simulink model "HANcoder_E407_TTA_Controller_v3"  (R2018b)
settings: Solver=FixedStepDiscrete  StartTime=0.0  StopTime=1  FixedStep=0.01  RelTol=1e-3
PreLoadFcn:
  | librarySetup
  | eval([bdroot,'_startup']) %Calling [modelName]_startup.m
values from neighbouring files (symbols this model uses):
  basic_cycle_duration_bc0 = TM_Reset_Board   + COMP_duration    (= 212)    [HANcoder_E407_TTA_Controller_v3_startup.m]
  basic_cycle_duration_bc1 = TM_Reset_Var_bc1 + COMP_duration    (= 288)    [HANcoder_E407_TTA_Controller_v3_startup.m]
  comm_delay_estimation1 = round(comm_delay_measured1*hardware_granularity/frequency_IRQ)    [HANcoder_E407_TTA_Controller_v3_startup.m]
  comm_delay_estimation2 = round(comm_delay_measured2*hardware_granularity/frequency_IRQ)    [HANcoder_E407_TTA_Controller_v3_startup.m]
  COMM_Period = 40    [HANcoder_E407_TTA_Controller_v3_startup.m]
  COMM_Phase1 = 5    [HANcoder_E407_TTA_Controller_v3_startup.m]
  COMM_Phase2 = 8    [HANcoder_E407_TTA_Controller_v3_startup.m]
  COMP_duration = 4    [HANcoder_E407_TTA_Controller_v3_startup.m]
  Controller1_Board = 1    [HANcoder_E407_TTA_Controller_v3_startup.m]
  Controller2_Board = 2    [HANcoder_E407_TTA_Controller_v3_startup.m]
  Controller3_Board = 3    [HANcoder_E407_TTA_Controller_v3_startup.m]
  delta_a_set = Simulink.Parameter    [HANcoder_E407_TTA_Controller_v3_startup.m]
  delta_f_set = Simulink.Parameter    [HANcoder_E407_TTA_Controller_v3_startup.m]
  delta_max = 1    [HANcoder_E407_TTA_Controller_v3_startup.m]
  delta_min = -1    [HANcoder_E407_TTA_Controller_v3_startup.m]
  delta_precision = 6    [HANcoder_E407_TTA_Controller_v3_startup.m]
  e_width = 0.1    [HANcoder_E407_TTA_Controller_v3_startup.m]
  frequency_IRQ = 100    [HANcoder_E407_TTA_Controller_v3_startup.m]
  HANtuneOverride = Simulink.Parameter    [HANcoder_E407_TTA_Controller_v3_startup.m]
  hardware_granularity = 1000000    [HANcoder_E407_TTA_Controller_v3_startup.m]
  I_a = 2.25    [HANcoder_E407_TTA_Controller_v3_startup.m]
  I_f = 2.25    [HANcoder_E407_TTA_Controller_v3_startup.m]
  idle_time_init = basic_cycle_duration_bc0 + basic_cycle_duration_bc1    (= 500)    [HANcoder_E407_TTA_Controller_v3_startup.m]
  Input_Gen_Board = 4    [HANcoder_E407_TTA_Controller_v3_startup.m]
  LA_Clock_Gr = 1    [HANcoder_E407_TTA_Controller_v3_startup.m]
  LA_COMM_Err = 0    [HANcoder_E407_TTA_Controller_v3_startup.m]
  LA_MEX_Flag = 0    [HANcoder_E407_TTA_Controller_v3_startup.m]
  LA_Task_Act = 1    [HANcoder_E407_TTA_Controller_v3_startup.m]
  m_v = 100.0    (= 100)    [HANcoder_E407_TTA_Controller_v3_startup.m]
  Master_Role = 1    [HANcoder_E407_TTA_Controller_v3_startup.m]
  matrix_cycle_duration = basic_cycle_duration_bc0 + basic_cycle_duration_bc1    (= 500)    [HANcoder_E407_TTA_Controller_v3_startup.m]
  matrix_rows = 2    [HANcoder_E407_TTA_Controller_v3_startup.m]
  max_num_msgs_CAN1 = 2^Tx_bit_number-1    (= 7)    [HANcoder_E407_TTA_Controller_v3_startup.m]
  max_num_msgs_CAN2 = max_num_msgs_CAN1    (= 7)    [HANcoder_E407_TTA_Controller_v3_startup.m]
  OutControl1_ID = 23    [HANcoder_E407_TTA_Controller_v3_startup.m]
  OutControl2_ID = 24    [HANcoder_E407_TTA_Controller_v3_startup.m]
  OutEmulator_ID = 25    [HANcoder_E407_TTA_Controller_v3_startup.m]
  R_al = 0.10    (= 0.1)    [HANcoder_E407_TTA_Controller_v3_startup.m]
  R_ar = 0.10    (= 0.1)    [HANcoder_E407_TTA_Controller_v3_startup.m]
  R_fl = 0.10    (= 0.1)    [HANcoder_E407_TTA_Controller_v3_startup.m]
  R_fr = 0.10    (= 0.1)    [HANcoder_E407_TTA_Controller_v3_startup.m]
  SensorValues_ID = 22    [HANcoder_E407_TTA_Controller_v3_startup.m]
  SetValues_ID = 21    [HANcoder_E407_TTA_Controller_v3_startup.m]
  Slave_Role = 2    [HANcoder_E407_TTA_Controller_v3_startup.m]
  speed_k_d = Simulink.Parameter    [HANcoder_E407_TTA_Controller_v3_startup.m]
  speed_k_i = Simulink.Parameter    [HANcoder_E407_TTA_Controller_v3_startup.m]
  speed_k_p = Simulink.Parameter    [HANcoder_E407_TTA_Controller_v3_startup.m]
  speed_max = 10    [HANcoder_E407_TTA_Controller_v3_startup.m]
  speed_min = -10    [HANcoder_E407_TTA_Controller_v3_startup.m]
  speed_precision = 3    [HANcoder_E407_TTA_Controller_v3_startup.m]
  Sync_ID = 1    [HANcoder_E407_TTA_Controller_v3_startup.m]
  tau_max = 5    [HANcoder_E407_TTA_Controller_v3_startup.m]
  tau_min = -5    [HANcoder_E407_TTA_Controller_v3_startup.m]
  tau_range = abs(tau_max) + abs(tau_min)    [HANcoder_E407_TTA_Controller_v3_startup.m]
  theta_max = 2    [HANcoder_E407_TTA_Controller_v3_startup.m]
  theta_min = -2    [HANcoder_E407_TTA_Controller_v3_startup.m]
  theta_precision = 5    [HANcoder_E407_TTA_Controller_v3_startup.m]
  Tl_a = 0.6    [HANcoder_E407_TTA_Controller_v3_startup.m]
  Tl_f = 0.6    [HANcoder_E407_TTA_Controller_v3_startup.m]
  TM_Check_Output_Control1 = TM_COMM_Output_Control1 + COMM_duration    (= 188)    [HANcoder_E407_TTA_Controller_v3_startup.m]
  TM_Check_Output_Control2 = TM_COMM_Output_Control2 + COMM_duration    (= 232)    [HANcoder_E407_TTA_Controller_v3_startup.m]
  TM_Check_Output_Emulator = TM_COMM_Output_Emulator + COMM_duration    (= 280)    [HANcoder_E407_TTA_Controller_v3_startup.m]
  TM_Check_Sensor_Values = TM_COMM_Sensor_Values + COMM_duration    (= 132)    [HANcoder_E407_TTA_Controller_v3_startup.m]
  TM_Check_Set_Values = TM_COMM_Set_Values + COMM_duration    (= 88)    [HANcoder_E407_TTA_Controller_v3_startup.m]
  TM_Check_Sync = TM_COMM_Sync   + COMM_duration    (= 40)    [HANcoder_E407_TTA_Controller_v3_startup.m]
  TM_Check_TOuts = TM_Count_Vote3 + COMP_duration    (= 196)    [HANcoder_E407_TTA_Controller_v3_startup.m]
  TM_Check_Vote1 = TM_COMM_Vote1  + COMM_duration    (= 92)    [HANcoder_E407_TTA_Controller_v3_startup.m]
  TM_Check_Vote2 = TM_COMM_Vote2  + COMM_duration    (= 140)    [HANcoder_E407_TTA_Controller_v3_startup.m]
  TM_Check_Vote3 = TM_COMM_Vote3  + COMM_duration    (= 188)    [HANcoder_E407_TTA_Controller_v3_startup.m]
  TM_COMM_Output_Control1 = TM_Velocity + COMP_duration    (= 148)    [HANcoder_E407_TTA_Controller_v3_startup.m]
  TM_COMM_Output_Control2 = TM_Check_Output_Control1 + COMP_duration    (= 192)    [HANcoder_E407_TTA_Controller_v3_startup.m]
  TM_COMM_Output_Emulator = TM_TMR + COMP_duration    (= 240)    [HANcoder_E407_TTA_Controller_v3_startup.m]
  TM_COMM_Sensor_Values = TM_Check_Set_Values + COMP_duration    (= 92)    [HANcoder_E407_TTA_Controller_v3_startup.m]
  TM_COMM_Set_Values = TM_Update_LT + COMP_duration    (= 48)    [HANcoder_E407_TTA_Controller_v3_startup.m]
  TM_COMM_Sync = basic_cycle_start    (= 0)    [HANcoder_E407_TTA_Controller_v3_startup.m]
  TM_COMM_Vote1 = TM_Vote_Dec    + COMP_duration    (= 52)    [HANcoder_E407_TTA_Controller_v3_startup.m]
  TM_COMM_Vote2 = TM_Count_Vote1 + COMP_duration    (= 100)    [HANcoder_E407_TTA_Controller_v3_startup.m]
  TM_COMM_Vote3 = TM_Count_Vote2 + COMP_duration    (= 148)    [HANcoder_E407_TTA_Controller_v3_startup.m]
  TM_Count_Vote1 = TM_Check_Vote1 + COMP_duration    (= 96)    [HANcoder_E407_TTA_Controller_v3_startup.m]
  TM_Count_Vote2 = TM_Check_Vote2 + COMP_duration    (= 144)    [HANcoder_E407_TTA_Controller_v3_startup.m]
  TM_Count_Vote3 = TM_Check_Vote3 + COMP_duration    (= 192)    [HANcoder_E407_TTA_Controller_v3_startup.m]
  TM_Data_bc0 = TM_COMM_Sync    (= 0)    [HANcoder_E407_TTA_Controller_v3_startup.m]
  TM_Data_bc1 = TM_Data_bc0(1:3)    [HANcoder_E407_TTA_Controller_v3_startup.m]
  TM_New_Master = TM_Check_TOuts + COMP_duration    (= 200)    [HANcoder_E407_TTA_Controller_v3_startup.m]
  TM_Reset_Board = TM_Reset_Var   + COMP_duration    (= 208)    [HANcoder_E407_TTA_Controller_v3_startup.m]
  TM_Reset_Var = TM_New_Master  + COMP_duration    (= 204)    [HANcoder_E407_TTA_Controller_v3_startup.m]
  TM_Reset_Var_bc1 = TM_Check_Output_Emulator + COMP_duration    (= 284)    [HANcoder_E407_TTA_Controller_v3_startup.m]
  TM_Steer = TM_Check_Sensor_Values + COMP_duration    (= 136)    [HANcoder_E407_TTA_Controller_v3_startup.m]
  TM_TMR = TM_Check_Output_Control2 + COMP_duration    (= 236)    [HANcoder_E407_TTA_Controller_v3_startup.m]
  TM_Torque = TM_Steer + COMP_duration    (= 140)    [HANcoder_E407_TTA_Controller_v3_startup.m]
  TM_Type_bc0 = COMM    (= 0)    [HANcoder_E407_TTA_Controller_v3_startup.m]
  TM_Type_bc1 = TM_Type_bc0(1:3)    [HANcoder_E407_TTA_Controller_v3_startup.m]
  TM_Update_LT = TM_Check_Sync  + COMP_duration    (= 44)    [HANcoder_E407_TTA_Controller_v3_startup.m]
  TM_Velocity = TM_Torque + COMP_duration    (= 144)    [HANcoder_E407_TTA_Controller_v3_startup.m]
  TM_Vote_Dec = TM_Update_LT   + COMP_duration    (= 48)    [HANcoder_E407_TTA_Controller_v3_startup.m]
  torque_a_k_d = Simulink.Parameter    [HANcoder_E407_TTA_Controller_v3_startup.m]
  torque_a_k_i = Simulink.Parameter    [HANcoder_E407_TTA_Controller_v3_startup.m]
  torque_a_k_p = Simulink.Parameter    [HANcoder_E407_TTA_Controller_v3_startup.m]
  torque_f_k_d = Simulink.Parameter    [HANcoder_E407_TTA_Controller_v3_startup.m]
  torque_f_k_i = Simulink.Parameter    [HANcoder_E407_TTA_Controller_v3_startup.m]
  torque_f_k_p = Simulink.Parameter    [HANcoder_E407_TTA_Controller_v3_startup.m]
  torque_precision = 4    [HANcoder_E407_TTA_Controller_v3_startup.m]
  v_set = Simulink.Parameter    [HANcoder_E407_TTA_Controller_v3_startup.m]
  Vehicle_Em_Board = 5    [HANcoder_E407_TTA_Controller_v3_startup.m]
  Vote1_ID = 11    [HANcoder_E407_TTA_Controller_v3_startup.m]
  Vote2_ID = 12    [HANcoder_E407_TTA_Controller_v3_startup.m]
  Vote3_ID = 13    [HANcoder_E407_TTA_Controller_v3_startup.m]
undefined symbols (not defined in the file or in its folder): A0, A1, A2, A3, A4, CON2
libraries: hdlsllib x352, HANcoder_STM32_Target x25, simulink x3, simulink_extras x1
(part 6 of 32)

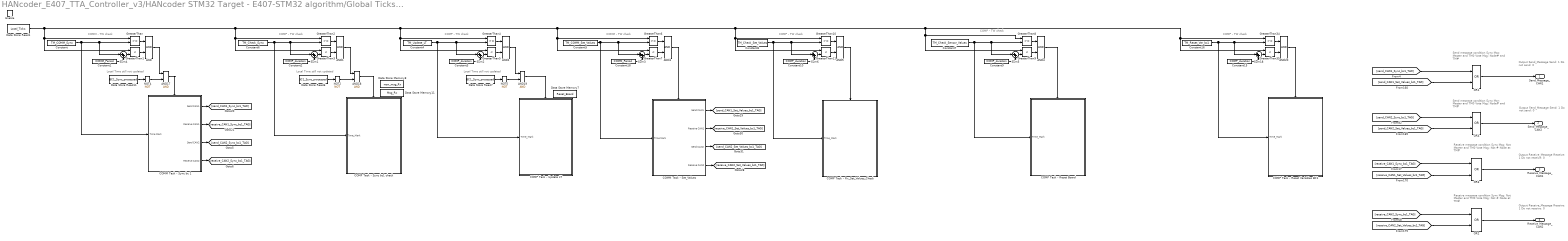
== system HANcoder_E407_TTA_Controller_v3/HANcoder STM32 Target - E407-STM32 algorithm/Global Ticks Increment/CAN Management/Matrix Cycle Manager/Input Generator Matrix Cycle/input generator basic cycle 1 ==
  note: COMP - TW check
  note: COMM - TW check
  note: Local Time still not updated
  note: Local Time still not updated
  note: COMP - TW check
  note: Local Time still not updated
  note: COMP - TW check
  note: COMP - TW check
  note: COMM - TW check
  note: Receive message condition
      | Sync Msg: Not Master and TM0
      | Vote Msg: Not # Node at TM#
  note: Send message condition
      | Sync Msg: Master and TM0
      | Vote Msg: Node# and TM#
  note: Output Send_Message
      | Send: 1
      | Do not send: 0
  note: Output Receive_Message
      | Receive: 1
      | Do not receive: 0
  note: Output Receive_Message
      | Receive: 1
      | Do not receive: 0
  note: Output Send_Message
      | Send: 1
      | Do not send: 0
  note: Send message condition
      | Sync Msg: Master and TM0
      | Vote Msg: Node# and TM#
  note: Receive message condition
      | Sync Msg: Not Master and TM0
      | Vote Msg: Not # Node at TM#
  note: COMP - TW check
  Enable : EnablePort
  AND{,1..5,17..20} (10 alike) : Logic  IconShape=distinctive  AllPortsSameDT=off  OutDataTypeStr=boolean
  COMM Task - Set_Values : Subsystem
  COMM Task - Sync bc 1 : Subsystem
  COMP Task - Reset Board : Subsystem
  COMP Task - Reset Variables BC1 : Subsystem
  COMP Task - Rx_Set_Values_Check : Subsystem
  COMP Task - Sync bc1 check : Subsystem
  COMP Task - Update LT : Subsystem
  Constant : Constant  Value=TM_COMM_Sync
  Constant1 : Constant  Value=COMM_Period
  Constant{2..3,9..10,15} (5 alike) : Constant  Value=COMP_duration
  Constant16 : Constant  Value=TM_Reset_Var_bc1
  Constant18 : Constant  Value=COMM_Period
  Constant4 : Constant  Value=TM_Update_LT
  Constant5 : Constant  Value=TM_COMM_Set_Values
  Constant6 : Constant  Value=TM_Check_Sync
  Constant7 : Constant  Value=TM_Check_Sensor_Values
  Constant8 : Constant  Value=TM_Check_Set_Values
  Data Store Memory11 : DataStoreMemory  DataStoreName=Msg_Rx  ReadBeforeWriteMsg=warning  WriteAfterWriteMsg=warning  WriteAfterReadMsg=warning  ShowAdditionalParam=off  OutDataTypeStr=Bus: msg_buffer_type
  Data Store Memory7 : DataStoreMemory  DataStoreName=Reset_Board  ReadBeforeWriteMsg=warning  WriteAfterWriteMsg=warning  WriteAfterReadMsg=warning  ShowAdditionalParam=off  OutDataTypeStr=boolean
  Data Store Memory8 : DataStoreMemory  DataStoreName=new_msg_Rx  ReadBeforeWriteMsg=warning  WriteAfterWriteMsg=warning  WriteAfterReadMsg=warning  ShowAdditionalParam=off
  Data Store Read1 : DataStoreRead  DataStoreName=Local_Ticks
  Data Store Read11 : DataStoreRead  DataStoreName=BC1_Sync_processed
  Data Store Read6 : DataStoreRead  DataStoreName=BC1_Sync_processed
  Data Store Read7 : DataStoreRead  DataStoreName=BC1_Sync_processed
  GreaterThan{,2,4,6,8,10,34} (7 alike) : RelationalOperator  OutDataTypeStr=boolean  RndMeth=Simplest
  GreaterThan{1,3,5,7,9,11,35} (7 alike) : RelationalOperator  Operator=<  OutDataTypeStr=boolean  RndMeth=Simplest
  NOT2 : Logic  Operator=NOT  IconShape=distinctive  AllPortsSameDT=off  OutDataTypeStr=boolean
  NOT4 : Logic  Operator=NOT  IconShape=distinctive  AllPortsSameDT=off  OutDataTypeStr=boolean
  NOT5 : Logic  Operator=NOT  IconShape=distinctive  AllPortsSameDT=off  OutDataTypeStr=boolean
  OR{1..4} (4 alike) : Logic  Operator=OR  IconShape=distinctive  AllPortsSameDT=off  OutDataTypeStr=boolean
  Sum{1..6,18} (7 alike) : Sum  Inputs=|++
  Send_Message_CAN1 : Outport  OutputWhenDisabled=reset  InitialOutput=0
  Send_Message_CAN2 : Outport  Port=2  OutputWhenDisabled=reset  InitialOutput=0
  Receive_Message_CAN1 : Outport  Port=3  OutputWhenDisabled=reset  InitialOutput=0
  Receive_Message_CAN2 : Outport  Port=4  OutputWhenDisabled=reset  InitialOutput=0
  wires:
  AND20/1 -> COMP Task - Reset Variables BC1/Enable
  GreaterThan34/1 -> AND20/1
  Sum18/1 -> GreaterThan35/2
  Constant15/1 -> Sum18/2
  Constant16/1 -> COMP Task - Reset Variables BC1/1(Time_Mark), GreaterThan34/2, Sum18/1
  GreaterThan35/1 -> AND20/2
  COMM Task - Set_Values/4(Receive CAN2) -> [receive_CAN2_Set_Values_bc1_TAG]
  COMM Task - Set_Values/3(Send CAN2) -> [send_CAN2_Set_Values_bc1_TAG]
  COMM Task - Set_Values/2(Receive CAN1) -> [receive_CAN1_Set_Values_bc1_TAG]
  COMM Task - Set_Values/1(Send CAN1) -> [send_CAN1_Set_Values_bc1_TAG]
  GreaterThan5/1 -> AND2/2
  Sum2/1 -> GreaterThan5/2
  NOT5/1 -> AND19/2
  COMM Task - Sync bc 1/3(Send CAN2) -> [send_CAN2_Sync_bc1_TAG]
  Sum1/1 -> GreaterThan3/2
  Constant6/1 -> Sum1/1, GreaterThan2/2, COMP Task - Sync bc1 check/1(Time_Mark)
  GreaterThan7/1 -> AND3/2
  Constant2/1 -> Sum1/2
  GreaterThan3/1 -> AND1/2
  GreaterThan2/1 -> AND1/1
  GreaterThan9/1 -> AND4/2
  GreaterThan8/1 -> AND4/1
  GreaterThan6/1 -> AND3/1
  Sum4/1 -> GreaterThan1/2
  Sum5/1 -> GreaterThan9/2
  Constant4/1 -> COMP Task - Update LT/1(Time_Mark), GreaterThan4/2, Sum2/1
  Sum3/1 -> GreaterThan7/2
  Constant7/1 -> COMP Task - Reset Board/1(Time_Mark), GreaterThan8/2, Sum5/1
  Constant3/1 -> Sum2/2
  AND/1 -> AND17/1
  Constant18/1 -> Sum3/2
  Constant5/1 -> Sum3/1, GreaterThan6/2, COMM Task - Set_Values/1(Time Mark)
  Constant/1 -> GreaterThan/2, Sum4/1, COMM Task - Sync bc 1/1(Time Mark)
  GreaterThan/1 -> AND/1
  GreaterThan1/1 -> AND/2
  NOT4/1 -> AND17/2
  Data Store Read6/1 -> NOT2/1
  AND2/1 -> AND19/1
  AND17/1 -> COMM Task - Sync bc 1/Enable
  Data Store Read11/1 -> NOT4/1
  AND1/1 -> AND18/1
  AND18/1 -> COMP Task - Sync bc1 check/Enable
  AND3/1 -> COMM Task - Set_Values/Enable
  GreaterThan4/1 -> AND2/1
  Data Store Read7/1 -> NOT5/1
  Constant9/1 -> Sum5/2
  NOT2/1 -> AND18/2
  AND4/1 -> COMP Task - Reset Board/Enable
  AND19/1 -> COMP Task - Update LT/Enable
  COMM Task - Sync bc 1/4(Receive CAN2) -> [receive_CAN2_Sync_bc1_TAG]
  COMM Task - Sync bc 1/2(Receive CAN1) -> [receive_CAN1_Sync_bc1_TAG]
  COMM Task - Sync bc 1/1(Send CAN1) -> [send_CAN1_Sync_bc1_TAG]
  Constant1/1 -> Sum4/2
  [receive_CAN2_Set_Values_bc1_TAG] -> OR2/2
  [receive_CAN2_Sync_bc1_TAG] -> OR2/1
  [receive_CAN1_Set_Values_bc1_TAG] -> OR3/2
  [receive_CAN1_Sync_bc1_TAG] -> OR3/1
  [send_CAN2_Set_Values_bc1_TAG] -> OR4/2
  [send_CAN2_Sync_bc1_TAG] -> OR4/1
  [send_CAN1_Set_Values_bc1_TAG] -> OR1/2
  [send_CAN1_Sync_bc1_TAG] -> OR1/1
  OR3/1 -> Receive_Message_CAN1/1
  OR4/1 -> Send_Message_CAN2/1
  OR2/1 -> Receive_Message_CAN2/1
  OR1/1 -> Send_Message_CAN1/1
  Constant8/1 -> COMP Task - Rx_Set_Values_Check/1(Time_Mark), Sum6/1, GreaterThan10/2
  GreaterThan10/1 -> AND5/1
  Data Store Read1/1 -> GreaterThan1/1, GreaterThan/1, GreaterThan3/1, GreaterThan2/1, GreaterThan5/1, GreaterThan4/1, GreaterThan7/1, GreaterThan6/1, GreaterThan35/1, GreaterThan34/1, GreaterThan9/1, GreaterThan8/1, GreaterThan11/1, GreaterThan10/1
  GreaterThan11/1 -> AND5/2
  Constant10/1 -> Sum6/2
  Sum6/1 -> GreaterThan11/2
  AND5/1 -> COMP Task - Rx_Set_Values_Check/Enable

== system HANcoder_E407_TTA_Controller_v3/HANcoder STM32 Target - E407-STM32 algorithm/Global Ticks Increment/CAN Management/Matrix Cycle Manager/Input Generator Matrix Cycle/msg_count_DEBUG observer ==
  Data Store Read24 : DataStoreRead  DataStoreName=msg_count_DEBUG
  Terminator : Terminator
  wires:
  Data Store Read24/1 -> Terminator/1  "msg_count_DEBUG_ing_s"

== system HANcoder_E407_TTA_Controller_v3/HANcoder STM32 Target - E407-STM32 algorithm/Global Ticks Increment/CAN Management/Matrix Cycle Manager/Vehicle Emulator Matrix Cycle/Matrix_Cycle_Observation_DEBUG ==
  Data Store Read : DataStoreRead  DataStoreName=Master_ID
  Data Store Read1 : DataStoreRead  DataStoreName=Role_ID
  Data Store Read10 : DataStoreRead  DataStoreName=BC1_Sync_processed
  Data Store Read2 : DataStoreRead  DataStoreName=BC0_Sync_processed
  Terminator{,1..2,12} (4 alike) : Terminator
  wires:
  Data Store Read1/1 -> Terminator/1  "Role_ID_vem_s"
  Data Store Read10/1 -> Terminator12/1  "BC1_sync_processed_vem__s"
  Data Store Read2/1 -> Terminator2/1  "BC0_sync_processed_vem__s"
  Data Store Read/1 -> Terminator1/1  "Master_ID_vem_s"

== system HANcoder_E407_TTA_Controller_v3/HANcoder STM32 Target - E407-STM32 algorithm/Global Ticks Increment/CAN Management/Matrix Cycle Manager/Vehicle Emulator Matrix Cycle/msg_count_DEBUG observer ==
  Data Store Read24 : DataStoreRead  DataStoreName=msg_count_DEBUG
  Terminator : Terminator
  wires:
  Data Store Read24/1 -> Terminator/1  "msg_count_DEBUG_vem_s"

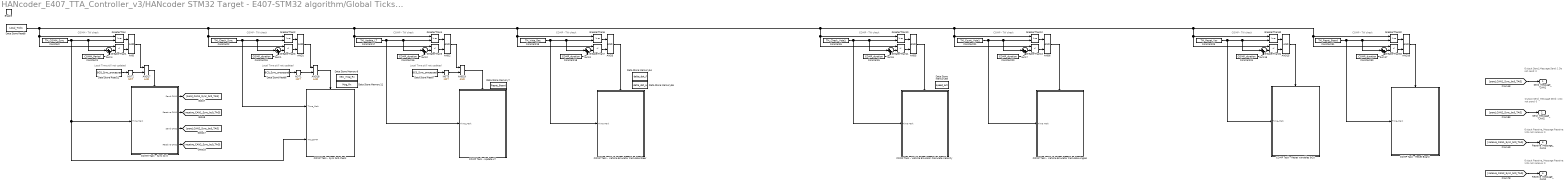
== system HANcoder_E407_TTA_Controller_v3/HANcoder STM32 Target - E407-STM32 algorithm/Global Ticks Increment/CAN Management/Matrix Cycle Manager/Vehicle Emulator Matrix Cycle/vehicle emulator basic cycle 0 ==
  note: Output Send_Message
      | Send: 1
      | Do not send: 0
  note: Output Receive_Message
      | Receive: 1
      | Do not receive: 0
  note: Output Send_Message
      | Send: 1
      | Do not send: 0
  note: Output Receive_Message
      | Receive: 1
      | Do not receive: 0
  note: COMM - TW check
  note: COMP - TW check
  note: COMP - TW check
  note: COMP - TW check
  note: COMP - TW check
  note: COMP - TW check
  note: COMP - TW check
  note: COMP - TW check
  note: Local Time still not updated
  note: Local Time still not updated
  note: Local Time still not updated
  Enable : EnablePort  PropagateVarSize=During execution
  AND{,1..3,5..6,15..19} (11 alike) : Logic  IconShape=distinctive  AllPortsSameDT=off  OutDataTypeStr=boolean
  COMM Task - Sync bc 0 : Subsystem
  COMP Task - Reset Board : Subsystem
  COMP Task - Reset Variables BC0 : Subsystem
  COMP Task - Sync bc0 check : Subsystem
  COMP Task - Update LT : Subsystem
  COMP Task - Vehicle Emulator Calculate Angles : Subsystem
  COMP Task - Vehicle Emulator Calculate Steer : Subsystem
  COMP Task - Vehicle Emulator Calculate Velocity : Subsystem
  Constant : Constant  Value=TM_COMM_Sync
  Constant1 : Constant  Value=COMM_Period
  Constant{5,15..16,18,20,24,30} (7 alike) : Constant  Value=COMP_duration
  Constant17 : Constant  Value=TM_Update_LT
  Constant19 : Constant  Value=TM_Vote_Dec
  Constant2 : Constant  Value=TM_Check_Sync
  Constant21 : Constant  Value=TM_Count_Vote1
  Constant25 : Constant  Value=TM_Reset_Var
  Constant31 : Constant  Value=TM_Reset_Board
  Constant6 : Constant  Value=TM_Check_Vote1
  Data Store Memory11 : DataStoreMemory  DataStoreName=Msg_Rx  ReadBeforeWriteMsg=warning  WriteAfterWriteMsg=warning  WriteAfterReadMsg=warning  ShowAdditionalParam=off  OutDataTypeStr=Bus: msg_buffer_type
  Data Store Memory54 : DataStoreMemory  DataStoreName=delta_dot_f  ReadBeforeWriteMsg=warning  WriteAfterWriteMsg=warning  WriteAfterReadMsg=warning  ShowAdditionalParam=off
  Data Store Memory56 : DataStoreMemory  DataStoreName=delta_dot_a  ReadBeforeWriteMsg=warning  WriteAfterWriteMsg=warning  WriteAfterReadMsg=warning  ShowAdditionalParam=off
  Data Store Memory59 : DataStoreMemory  DataStoreName=speed_act  ReadBeforeWriteMsg=warning  WriteAfterWriteMsg=warning  WriteAfterReadMsg=warning  ShowAdditionalParam=off
  Data Store Memory7 : DataStoreMemory  DataStoreName=Reset_Board  ReadBeforeWriteMsg=warning  WriteAfterWriteMsg=warning  WriteAfterReadMsg=warning  ShowAdditionalParam=off  OutDataTypeStr=boolean
  Data Store Memory8 : DataStoreMemory  DataStoreName=new_msg_Rx  ReadBeforeWriteMsg=warning  WriteAfterWriteMsg=warning  WriteAfterReadMsg=warning  ShowAdditionalParam=off
  Data Store Read11 : DataStoreRead  DataStoreName=BC0_Sync_processed
  Data Store Read6 : DataStoreRead  DataStoreName=BC0_Sync_processed
  Data Store Read7 : DataStoreRead  DataStoreName=BC0_Sync_processed
  Data Store Read8 : DataStoreRead  DataStoreName=Local_Ticks
  GreaterThan{,2,4,6,10,12,30,32} (8 alike) : RelationalOperator  OutDataTypeStr=boolean  RndMeth=Simplest
  GreaterThan{1,3,5,7,11,13,31,33} (8 alike) : RelationalOperator  Operator=<  OutDataTypeStr=boolean  RndMeth=Simplest
  NOT1 : Logic  Operator=NOT  IconShape=distinctive  AllPortsSameDT=off  OutDataTypeStr=boolean
  NOT2 : Logic  Operator=NOT  IconShape=distinctive  AllPortsSameDT=off  OutDataTypeStr=boolean
  NOT3 : Logic  Operator=NOT  IconShape=distinctive  AllPortsSameDT=off  OutDataTypeStr=boolean
  Sum{1..4,6..7,16..17} (8 alike) : Sum  Inputs=|++
  Send_Message_CAN1 : Outport  OutputWhenDisabled=reset  InitialOutput=0
  Send_Message_CAN2 : Outport  Port=2  OutputWhenDisabled=reset  InitialOutput=0
  Receive_Message_CAN1 : Outport  Port=3  OutputWhenDisabled=reset  InitialOutput=0
  Receive_Message_CAN2 : Outport  Port=4  OutputWhenDisabled=reset  InitialOutput=0
  wires:
  COMM Task - Sync bc 0/1(Send CAN1) -> [send_CAN1_Sync_bc0_TAG]
  COMM Task - Sync bc 0/2(Receive CAN1) -> [receive_CAN1_Sync_bc0_TAG]
  COMM Task - Sync bc 0/3(Send CAN2) -> [send_CAN2_Sync_bc0_TAG]
  COMM Task - Sync bc 0/4(Receive CAN2) -> [receive_CAN2_Sync_bc0_TAG]
  Constant1/1 -> Sum4/2
  Constant/1 -> COMP Task - Sync bc0 check/2(TM_COMM), COMM Task - Sync bc 0/1(Time Mark), Sum4/1, GreaterThan/2
  Sum4/1 -> GreaterThan1/2
  GreaterThan/1 -> AND/1
  GreaterThan1/1 -> AND/2
  AND/1 -> AND17/1
  GreaterThan3/1 -> AND1/2
  GreaterThan2/1 -> AND1/1
  Sum1/1 -> GreaterThan3/2
  Constant2/1 -> COMP Task - Sync bc0 check/1(Time_Mark), GreaterThan2/2, Sum1/1
  Constant15/1 -> Sum1/2
  Constant16/1 -> Sum2/2
  Constant17/1 -> COMP Task - Update LT/1(Time_Mark), Sum2/1, GreaterThan4/2
  Sum2/1 -> GreaterThan5/2
  GreaterThan4/1 -> AND2/1
  GreaterThan5/1 -> AND2/2
  AND3/1 -> COMP Task - Vehicle Emulator Calculate Steer/Enable
  GreaterThan7/1 -> AND3/2
  GreaterThan6/1 -> AND3/1
  Sum3/1 -> GreaterThan7/2
  Constant19/1 -> COMP Task - Vehicle Emulator Calculate Steer/1(Time Mark), GreaterThan6/2, Sum3/1
  Constant18/1 -> Sum3/2
  GreaterThan11/1 -> AND5/2
  Sum6/1 -> GreaterThan11/2
  GreaterThan10/1 -> AND5/1
  Constant5/1 -> Sum6/2
  Constant6/1 -> COMP Task - Vehicle Emulator Calculate Velocity/1(Time Mark), GreaterThan10/2, Sum6/1
  AND5/1 -> COMP Task - Vehicle Emulator Calculate Velocity/Enable
  AND6/1 -> COMP Task - Vehicle Emulator Calculate Angles/Enable
  Constant21/1 -> COMP Task - Vehicle Emulator Calculate Angles/1(Time Mark), Sum7/1, GreaterThan12/2
  Constant20/1 -> Sum7/2
  GreaterThan12/1 -> AND6/1
  Sum7/1 -> GreaterThan13/2
  GreaterThan13/1 -> AND6/2
  GreaterThan31/1 -> AND15/2
  Sum16/1 -> GreaterThan31/2
  GreaterThan30/1 -> AND15/1
  Constant24/1 -> Sum16/2
  Constant25/1 -> COMP Task - Reset Variables BC0/1(Time_Mark), GreaterThan30/2, Sum16/1
  AND15/1 -> COMP Task - Reset Variables BC0/Enable
  Data Store Read8/1 -> GreaterThan32/1, GreaterThan33/1, GreaterThan31/1, GreaterThan30/1, GreaterThan12/1, GreaterThan13/1, GreaterThan11/1, GreaterThan10/1, GreaterThan6/1, GreaterThan7/1, GreaterThan4/1, GreaterThan5/1, GreaterThan2/1, GreaterThan3/1, GreaterThan/1, GreaterThan1/1
  AND16/1 -> COMP Task - Reset Board/Enable
  Constant31/1 -> COMP Task - Reset Board/1(Time_Mark), Sum17/1, GreaterThan32/2
  Constant30/1 -> Sum17/2
  GreaterThan32/1 -> AND16/1
  Sum17/1 -> GreaterThan33/2
  GreaterThan33/1 -> AND16/2
  Data Store Read11/1 -> NOT2/1
  NOT2/1 -> AND17/2
  AND17/1 -> COMM Task - Sync bc 0/Enable
  Data Store Read6/1 -> NOT1/1
  NOT1/1 -> AND18/2
  AND1/1 -> AND18/1
  AND18/1 -> COMP Task - Sync bc0 check/Enable
  Data Store Read7/1 -> NOT3/1
  NOT3/1 -> AND19/2
  AND2/1 -> AND19/1
  AND19/1 -> COMP Task - Update LT/Enable
  [send_CAN2_Sync_bc0_TAG] -> Send_Message_CAN2/1
  [receive_CAN1_Sync_bc0_TAG] -> Receive_Message_CAN1/1
  [receive_CAN2_Sync_bc0_TAG] -> Receive_Message_CAN2/1
  [send_CAN1_Sync_bc0_TAG] -> Send_Message_CAN1/1

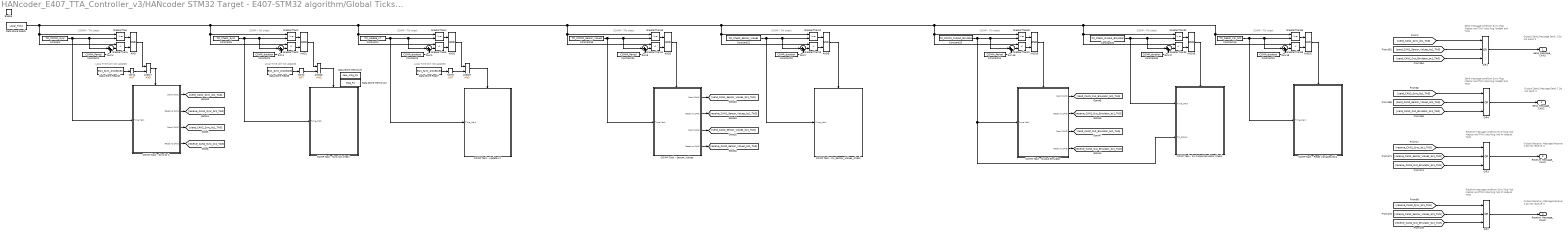
== system HANcoder_E407_TTA_Controller_v3/HANcoder STM32 Target - E407-STM32 algorithm/Global Ticks Increment/CAN Management/Matrix Cycle Manager/Vehicle Emulator Matrix Cycle/vehicle emulator basic cycle 1 ==
  note: Receive message condition
      | Sync Msg: Not Master and TM0
      | Vote Msg: Not # Node at TM#
  note: Send message condition
      | Sync Msg: Master and TM0
      | Vote Msg: Node# and TM#
  note: Output Send_Message
      | Send: 1
      | Do not send: 0
  note: Output Receive_Message
      | Receive: 1
      | Do not receive: 0
  note: Output Receive_Message
      | Receive: 1
      | Do not receive: 0
  note: Output Send_Message
      | Send: 1
      | Do not send: 0
  note: Send message condition
      | Sync Msg: Master and TM0
      | Vote Msg: Node# and TM#
  note: Receive message condition
      | Sync Msg: Not Master and TM0
      | Vote Msg: Not # Node at TM#
  note: COMM - TW check
  note: COMP - TW check
  note: COMM - TW check
  note: COMP - TW check
  note: Local Time still not updated
  note: COMP - TW check
  note: Local Time still not updated
  note: COMP - TW check
  note: Local Time still not updated
  note: COMP - TW check
  note: COMP - TW check
  Enable : EnablePort
  AND{,1..2,5..6,15..20} (11 alike) : Logic  IconShape=distinctive  AllPortsSameDT=off  OutDataTypeStr=boolean
  COMM Task - Output Emulator : Subsystem
  COMM Task - Sensor_Values : Subsystem
  COMM Task - Sync bc 1 : Subsystem
  COMP Task - Reset Variables BC1 : Subsystem
  COMP Task - Rx Output Emulator Check : Subsystem
  COMP Task - Rx_Sensor_Values_Check : Subsystem
  COMP Task - Sync bc1 check : Subsystem
  COMP Task - Update LT : Subsystem
  Constant : Constant  Value=TM_COMM_Sync
  Constant1 : Constant  Value=COMM_Period
  Constant{2..3,15,20,30} (5 alike) : Constant  Value=COMP_duration
  Constant16 : Constant  Value=TM_Reset_Var_bc1
  Constant21 : Constant  Value=TM_Check_Sensor_Values
  Constant24 : Constant  Value=COMM_Period
  Constant25 : Constant  Value=TM_COMM_Output_Emulator
  Constant31 : Constant  Value=TM_Check_Output_Emulator
  Constant34 : Constant  Value=COMM_Period
  Constant35 : Constant  Value=TM_COMM_Sensor_Values
  Constant4 : Constant  Value=TM_Update_LT
  Constant6 : Constant  Value=TM_Check_Sync
  Data Store Memory11 : DataStoreMemory  DataStoreName=Msg_Rx  ReadBeforeWriteMsg=warning  WriteAfterWriteMsg=warning  WriteAfterReadMsg=warning  ShowAdditionalParam=off  OutDataTypeStr=Bus: msg_buffer_type
  Data Store Memory8 : DataStoreMemory  DataStoreName=new_msg_Rx  ReadBeforeWriteMsg=warning  WriteAfterWriteMsg=warning  WriteAfterReadMsg=warning  ShowAdditionalParam=off
  Data Store Read1 : DataStoreRead  DataStoreName=Local_Ticks
  Data Store Read11 : DataStoreRead  DataStoreName=BC1_Sync_processed
  Data Store Read6 : DataStoreRead  DataStoreName=BC1_Sync_processed
  Data Store Read7 : DataStoreRead  DataStoreName=BC1_Sync_processed
  GreaterThan{,2,4,10,12,30,32,34} (8 alike) : RelationalOperator  OutDataTypeStr=boolean  RndMeth=Simplest
  GreaterThan{1,3,5,11,13,31,33,35} (8 alike) : RelationalOperator  Operator=<  OutDataTypeStr=boolean  RndMeth=Simplest
  NOT2 : Logic  Operator=NOT  IconShape=distinctive  AllPortsSameDT=off  OutDataTypeStr=boolean
  NOT4 : Logic  Operator=NOT  IconShape=distinctive  AllPortsSameDT=off  OutDataTypeStr=boolean
  NOT5 : Logic  Operator=NOT  IconShape=distinctive  AllPortsSameDT=off  OutDataTypeStr=boolean
  OR{1..4} (4 alike) : Logic  Operator=OR  Inputs=3  IconShape=distinctive  AllPortsSameDT=off  OutDataTypeStr=boolean
  Sum{1..2,4,6..7,16..18} (8 alike) : Sum  Inputs=|++
  Send_Message_CAN1 : Outport  OutputWhenDisabled=reset  InitialOutput=0
  Send_Message_CAN2 : Outport  Port=2  OutputWhenDisabled=reset  InitialOutput=0
  Receive_Message_CAN1 : Outport  Port=3  OutputWhenDisabled=reset  InitialOutput=0
  Receive_Message_CAN2 : Outport  Port=4  OutputWhenDisabled=reset  InitialOutput=0
  wires:
  COMM Task - Sensor_Values/3(Send CAN2) -> [send_CAN2_Sensor_Values_bc1_TAG]
  COMM Task - Sensor_Values/1(Send CAN1) -> [send_CAN1_Sensor_Values_bc1_TAG]
  COMM Task - Sensor_Values/2(Receive CAN1) -> [receive_CAN1_Sensor_Values_bc1_TAG]
  COMM Task - Sensor_Values/4(Receive CAN2) -> [receive_CAN2_Sensor_Values_bc1_TAG]
  OR1/1 -> Send_Message_CAN1/1
  OR2/1 -> Receive_Message_CAN2/1
  OR4/1 -> Send_Message_CAN2/1
  OR3/1 -> Receive_Message_CAN1/1
  [send_CAN1_Sync_bc1_TAG] -> OR1/1
  [send_CAN1_Sensor_Values_bc1_TAG] -> OR1/2
  [send_CAN1_Out_Emulator_bc1_TAG] -> OR1/3
  [send_CAN2_Sync_bc1_TAG] -> OR4/1
  [send_CAN2_Sensor_Values_bc1_TAG] -> OR4/2
  [send_CAN2_Out_Emulator_bc1_TAG] -> OR4/3
  [receive_CAN1_Sync_bc1_TAG] -> OR3/1
  [receive_CAN1_Sensor_Values_bc1_TAG] -> OR3/2
  [receive_CAN1_Out_Emulator_bc1_TAG] -> OR3/3
  [receive_CAN2_Sync_bc1_TAG] -> OR2/1
  [receive_CAN2_Sensor_Values_bc1_TAG] -> OR2/2
  [receive_CAN2_Out_Emulator_bc1_TAG] -> OR2/3
  Constant1/1 -> Sum4/2
  COMM Task - Sync bc 1/1(Send CAN1) -> [send_CAN1_Sync_bc1_TAG]
  COMM Task - Sync bc 1/2(Receive CAN1) -> [receive_CAN1_Sync_bc1_TAG]
  COMM Task - Sync bc 1/4(Receive CAN2) -> [receive_CAN2_Sync_bc1_TAG]
  AND19/1 -> COMP Task - Update LT/Enable
  NOT2/1 -> AND18/2
  Data Store Read7/1 -> NOT5/1
  GreaterThan4/1 -> AND2/1
  Constant31/1 -> COMP Task - Rx Output Emulator Check/1(Time_Mark), Sum17/1, GreaterThan32/2
  AND18/1 -> COMP Task - Sync bc1 check/Enable
  AND1/1 -> AND18/1
  Sum17/1 -> GreaterThan33/2
  Constant30/1 -> Sum17/2
  Data Store Read11/1 -> NOT4/1
  AND17/1 -> COMM Task - Sync bc 1/Enable
  GreaterThan33/1 -> AND16/2
  AND2/1 -> AND19/1
  GreaterThan32/1 -> AND16/1
  Data Store Read6/1 -> NOT2/1
  NOT4/1 -> AND17/2
  AND15/1 -> COMM Task - Output Emulator/Enable
  AND16/1 -> COMP Task - Rx Output Emulator Check/Enable
  GreaterThan30/1 -> AND15/1
  Sum16/1 -> GreaterThan31/2
  Constant24/1 -> Sum16/2
  Constant25/1 -> COMP Task - Rx Output Emulator Check/2(TM_COMM), COMM Task - Output Emulator/1(Time Mark), GreaterThan30/2, Sum16/1
  GreaterThan1/1 -> AND/2
  GreaterThan/1 -> AND/1
  GreaterThan10/1 -> AND5/1
  Constant/1 -> COMM Task - Sync bc 1/1(Time Mark), Sum4/1, GreaterThan/2
  AND/1 -> AND17/1
  Sum6/1 -> GreaterThan11/2
  Constant3/1 -> Sum2/2
  Constant35/1 -> COMM Task - Sensor_Values/1(Time Mark), GreaterThan10/2, Sum6/1
  Constant4/1 -> COMP Task - Update LT/1(Time_Mark), Sum2/1, GreaterThan4/2
  Sum4/1 -> GreaterThan1/2
  AND5/1 -> COMM Task - Sensor_Values/Enable
  GreaterThan31/1 -> AND15/2
  GreaterThan2/1 -> AND1/1
  GreaterThan3/1 -> AND1/2
  Constant2/1 -> Sum1/2
  Constant6/1 -> COMP Task - Sync bc1 check/1(Time_Mark), GreaterThan2/2, Sum1/1
  GreaterThan11/1 -> AND5/2
  Sum1/1 -> GreaterThan3/2
  Constant34/1 -> Sum6/2
  COMM Task - Sync bc 1/3(Send CAN2) -> [send_CAN2_Sync_bc1_TAG]
  NOT5/1 -> AND19/2
  Sum2/1 -> GreaterThan5/2
  GreaterThan5/1 -> AND2/2
  GreaterThan35/1 -> AND20/2
  Constant16/1 -> Sum18/1, GreaterThan34/2, COMP Task - Reset Variables BC1/1(Time_Mark)
  Constant15/1 -> Sum18/2
  Sum18/1 -> GreaterThan35/2
  GreaterThan34/1 -> AND20/1
  AND20/1 -> COMP Task - Reset Variables BC1/Enable
  COMM Task - Output Emulator/1(Send CAN1) -> [send_CAN1_Out_Emulator_bc1_TAG]
  COMM Task - Output Emulator/2(Receive CAN1) -> [receive_CAN1_Out_Emulator_bc1_TAG]
  COMM Task - Output Emulator/3(Send CAN2) -> [send_CAN2_Out_Emulator_bc1_TAG]
  COMM Task - Output Emulator/4(Receive CAN2) -> [receive_CAN2_Out_Emulator_bc1_TAG]
  GreaterThan13/1 -> AND6/2
  Data Store Read1/1 -> GreaterThan30/1, GreaterThan31/1, GreaterThan34/1, GreaterThan35/1, GreaterThan32/1, GreaterThan33/1, GreaterThan12/1, GreaterThan13/1, GreaterThan11/1, GreaterThan10/1, GreaterThan4/1, GreaterThan5/1, GreaterThan2/1, GreaterThan3/1, GreaterThan/1, GreaterThan1/1
  Constant21/1 -> COMP Task - Rx_Sensor_Values_Check/1(Time_Mark), Sum7/1, GreaterThan12/2
  AND6/1 -> COMP Task - Rx_Sensor_Values_Check/Enable
  Constant20/1 -> Sum7/2
  GreaterThan12/1 -> AND6/1
  Sum7/1 -> GreaterThan13/2

== system HANcoder_E407_TTA_Controller_v3/HANcoder STM32 Target - E407-STM32 algorithm/Global Ticks Increment/CAN1 Recieve/RxID_CAN/OutControl1_ID_CAN/CAN receive1 ==
  In1 : Inport
  Enabled Subsystem : Subsystem  TreatAsAtomicUnit=on
  S-Function : M-S-Function  FunctionName=sfcn_can_receive  Parameters=tsamp, canBus, outputNumber, dataType, byteOrder
  Out1 : Outport
  Out2 : Outport  Port=2
  Out3 : Outport  Port=3
  Out4 : Outport  Port=4
  Out5 : Outport  Port=5
  Out6 : Outport  Port=6
  Out7 : Outport  Port=7
  Out8 : Outport  Port=8
  Out9 : Outport  Port=9
  wires:
  S-Function/9 -> Enabled Subsystem/8(In8)
  S-Function/4 -> Enabled Subsystem/3(In3)
  S-Function/5 -> Enabled Subsystem/4(In4)
  S-Function/8 -> Enabled Subsystem/7(In7)
  S-Function/7 -> Enabled Subsystem/6(In6)
  S-Function/6 -> Enabled Subsystem/5(In5)
  Enabled Subsystem/8(Out8) -> Out9/1
  Enabled Subsystem/7(Out7) -> Out8/1
  Enabled Subsystem/6(Out6) -> Out7/1
  Enabled Subsystem/5(Out5) -> Out6/1
  Enabled Subsystem/4(Out4) -> Out5/1
  Enabled Subsystem/3(Out3) -> Out4/1
  Enabled Subsystem/2(Out2) -> Out3/1
  Enabled Subsystem/1(Out1) -> Out2/1
  S-Function/3 -> Enabled Subsystem/2(In2)
  S-Function/2 -> Enabled Subsystem/1(In1)
  S-Function/1 -> Out1/1, Enabled Subsystem/Enable
  In1/1 -> S-Function/1

== system HANcoder_E407_TTA_Controller_v3/HANcoder STM32 Target - E407-STM32 algorithm/Global Ticks Increment/CAN1 Recieve/RxID_CAN/OutControl2_ID_CAN/CAN receive1 ==
  In1 : Inport
  Enabled Subsystem : Subsystem  TreatAsAtomicUnit=on
  S-Function : M-S-Function  FunctionName=sfcn_can_receive  Parameters=tsamp, canBus, outputNumber, dataType, byteOrder
  Out1 : Outport
  Out2 : Outport  Port=2
  Out3 : Outport  Port=3
  Out4 : Outport  Port=4
  Out5 : Outport  Port=5
  Out6 : Outport  Port=6
  Out7 : Outport  Port=7
  Out8 : Outport  Port=8
  Out9 : Outport  Port=9
  wires:
  In1/1 -> S-Function/1
  S-Function/1 -> Enabled Subsystem/Enable, Out1/1
  S-Function/2 -> Enabled Subsystem/1(In1)
  S-Function/3 -> Enabled Subsystem/2(In2)
  Enabled Subsystem/1(Out1) -> Out2/1
  Enabled Subsystem/2(Out2) -> Out3/1
  Enabled Subsystem/3(Out3) -> Out4/1
  Enabled Subsystem/4(Out4) -> Out5/1
  Enabled Subsystem/5(Out5) -> Out6/1
  Enabled Subsystem/6(Out6) -> Out7/1
  Enabled Subsystem/7(Out7) -> Out8/1
  Enabled Subsystem/8(Out8) -> Out9/1
  S-Function/6 -> Enabled Subsystem/5(In5)
  S-Function/7 -> Enabled Subsystem/6(In6)
  S-Function/8 -> Enabled Subsystem/7(In7)
  S-Function/5 -> Enabled Subsystem/4(In4)
  S-Function/4 -> Enabled Subsystem/3(In3)
  S-Function/9 -> Enabled Subsystem/8(In8)

== system HANcoder_E407_TTA_Controller_v3/HANcoder STM32 Target - E407-STM32 algorithm/Global Ticks Increment/CAN1 Recieve/RxID_CAN/OutEmulator_ID_CAN/CAN receive1 ==
  In1 : Inport
  Enabled Subsystem : Subsystem  TreatAsAtomicUnit=on
  S-Function : M-S-Function  FunctionName=sfcn_can_receive  Parameters=tsamp, canBus, outputNumber, dataType, byteOrder
  Out1 : Outport
  Out2 : Outport  Port=2
  Out3 : Outport  Port=3
  Out4 : Outport  Port=4
  Out5 : Outport  Port=5
  Out6 : Outport  Port=6
  Out7 : Outport  Port=7
  Out8 : Outport  Port=8
  Out9 : Outport  Port=9
  wires:
  S-Function/9 -> Enabled Subsystem/8(In8)
  S-Function/4 -> Enabled Subsystem/3(In3)
  S-Function/5 -> Enabled Subsystem/4(In4)
  S-Function/8 -> Enabled Subsystem/7(In7)
  S-Function/7 -> Enabled Subsystem/6(In6)
  S-Function/6 -> Enabled Subsystem/5(In5)
  Enabled Subsystem/8(Out8) -> Out9/1
  Enabled Subsystem/7(Out7) -> Out8/1
  Enabled Subsystem/6(Out6) -> Out7/1
  Enabled Subsystem/5(Out5) -> Out6/1
  Enabled Subsystem/4(Out4) -> Out5/1
  Enabled Subsystem/3(Out3) -> Out4/1
  Enabled Subsystem/2(Out2) -> Out3/1
  Enabled Subsystem/1(Out1) -> Out2/1
  S-Function/3 -> Enabled Subsystem/2(In2)
  S-Function/2 -> Enabled Subsystem/1(In1)
  S-Function/1 -> Out1/1, Enabled Subsystem/Enable
  In1/1 -> S-Function/1

== system HANcoder_E407_TTA_Controller_v3/HANcoder STM32 Target - E407-STM32 algorithm/Global Ticks Increment/CAN1 Recieve/RxID_CAN/SensorValues_ID_CAN/CAN receive1 ==
  In1 : Inport
  Enabled Subsystem : Subsystem  TreatAsAtomicUnit=on
  S-Function : M-S-Function  FunctionName=sfcn_can_receive  Parameters=tsamp, canBus, outputNumber, dataType, byteOrder
  Out1 : Outport
  Out2 : Outport  Port=2
  Out3 : Outport  Port=3
  Out4 : Outport  Port=4
  Out5 : Outport  Port=5
  Out6 : Outport  Port=6
  Out7 : Outport  Port=7
  Out8 : Outport  Port=8
  Out9 : Outport  Port=9
  wires:
  In1/1 -> S-Function/1
  S-Function/1 -> Enabled Subsystem/Enable, Out1/1
  S-Function/2 -> Enabled Subsystem/1(In1)
  S-Function/3 -> Enabled Subsystem/2(In2)
  Enabled Subsystem/1(Out1) -> Out2/1
  Enabled Subsystem/2(Out2) -> Out3/1
  Enabled Subsystem/3(Out3) -> Out4/1
  Enabled Subsystem/4(Out4) -> Out5/1
  Enabled Subsystem/5(Out5) -> Out6/1
  Enabled Subsystem/6(Out6) -> Out7/1
  Enabled Subsystem/7(Out7) -> Out8/1
  Enabled Subsystem/8(Out8) -> Out9/1
  S-Function/6 -> Enabled Subsystem/5(In5)
  S-Function/7 -> Enabled Subsystem/6(In6)
  S-Function/8 -> Enabled Subsystem/7(In7)
  S-Function/5 -> Enabled Subsystem/4(In4)
  S-Function/4 -> Enabled Subsystem/3(In3)
  S-Function/9 -> Enabled Subsystem/8(In8)

== system HANcoder_E407_TTA_Controller_v3/HANcoder STM32 Target - E407-STM32 algorithm/Global Ticks Increment/CAN1 Recieve/RxID_CAN/SetValues_ID_CAN/CAN receive1 ==
  In1 : Inport
  Enabled Subsystem : Subsystem  TreatAsAtomicUnit=on
  S-Function : M-S-Function  FunctionName=sfcn_can_receive  Parameters=tsamp, canBus, outputNumber, dataType, byteOrder
  Out1 : Outport
  Out2 : Outport  Port=2
  Out3 : Outport  Port=3
  Out4 : Outport  Port=4
  Out5 : Outport  Port=5
  Out6 : Outport  Port=6
  Out7 : Outport  Port=7
  Out8 : Outport  Port=8
  Out9 : Outport  Port=9
  wires:
  S-Function/9 -> Enabled Subsystem/8(In8)
  S-Function/4 -> Enabled Subsystem/3(In3)
  S-Function/5 -> Enabled Subsystem/4(In4)
  S-Function/8 -> Enabled Subsystem/7(In7)
  S-Function/7 -> Enabled Subsystem/6(In6)
  S-Function/6 -> Enabled Subsystem/5(In5)
  Enabled Subsystem/8(Out8) -> Out9/1
  Enabled Subsystem/7(Out7) -> Out8/1
  Enabled Subsystem/6(Out6) -> Out7/1
  Enabled Subsystem/5(Out5) -> Out6/1
  Enabled Subsystem/4(Out4) -> Out5/1
  Enabled Subsystem/3(Out3) -> Out4/1
  Enabled Subsystem/2(Out2) -> Out3/1
  Enabled Subsystem/1(Out1) -> Out2/1
  S-Function/3 -> Enabled Subsystem/2(In2)
  S-Function/2 -> Enabled Subsystem/1(In1)
  S-Function/1 -> Out1/1, Enabled Subsystem/Enable
  In1/1 -> S-Function/1

== system HANcoder_E407_TTA_Controller_v3/HANcoder STM32 Target - E407-STM32 algorithm/Global Ticks Increment/CAN1 Recieve/RxID_CAN/Sync_ID_CAN/CAN receive1 ==
  In1 : Inport
  Enabled Subsystem : Subsystem  TreatAsAtomicUnit=on
  S-Function : M-S-Function  FunctionName=sfcn_can_receive  Parameters=tsamp, canBus, outputNumber, dataType, byteOrder
  Out1 : Outport
  Out2 : Outport  Port=2
  Out3 : Outport  Port=3
  Out4 : Outport  Port=4
  Out5 : Outport  Port=5
  Out6 : Outport  Port=6
  Out7 : Outport  Port=7
  Out8 : Outport  Port=8
  Out9 : Outport  Port=9
  wires:
  S-Function/9 -> Enabled Subsystem/8(In8)
  S-Function/4 -> Enabled Subsystem/3(In3)
  S-Function/5 -> Enabled Subsystem/4(In4)
  S-Function/8 -> Enabled Subsystem/7(In7)
  S-Function/7 -> Enabled Subsystem/6(In6)
  S-Function/6 -> Enabled Subsystem/5(In5)
  Enabled Subsystem/8(Out8) -> Out9/1
  Enabled Subsystem/7(Out7) -> Out8/1
  Enabled Subsystem/6(Out6) -> Out7/1
  Enabled Subsystem/5(Out5) -> Out6/1
  Enabled Subsystem/4(Out4) -> Out5/1
  Enabled Subsystem/3(Out3) -> Out4/1
  Enabled Subsystem/2(Out2) -> Out3/1
  Enabled Subsystem/1(Out1) -> Out2/1
  S-Function/3 -> Enabled Subsystem/2(In2)
  S-Function/2 -> Enabled Subsystem/1(In1)
  S-Function/1 -> Out1/1, Enabled Subsystem/Enable
  In1/1 -> S-Function/1

== system HANcoder_E407_TTA_Controller_v3/HANcoder STM32 Target - E407-STM32 algorithm/Global Ticks Increment/CAN1 Recieve/RxID_CAN/Vote1_ID_CAN/CAN receive1 ==
  In1 : Inport
  Enabled Subsystem : Subsystem  TreatAsAtomicUnit=on
  S-Function : M-S-Function  FunctionName=sfcn_can_receive  Parameters=tsamp, canBus, outputNumber, dataType, byteOrder
  Out1 : Outport
  Out2 : Outport  Port=2
  Out3 : Outport  Port=3
  Out4 : Outport  Port=4
  Out5 : Outport  Port=5
  Out6 : Outport  Port=6
  Out7 : Outport  Port=7
  Out8 : Outport  Port=8
  Out9 : Outport  Port=9
  wires:
  In1/1 -> S-Function/1
  S-Function/1 -> Enabled Subsystem/Enable, Out1/1
  S-Function/2 -> Enabled Subsystem/1(In1)
  S-Function/3 -> Enabled Subsystem/2(In2)
  Enabled Subsystem/1(Out1) -> Out2/1
  Enabled Subsystem/2(Out2) -> Out3/1
  Enabled Subsystem/3(Out3) -> Out4/1
  Enabled Subsystem/4(Out4) -> Out5/1
  Enabled Subsystem/5(Out5) -> Out6/1
  Enabled Subsystem/6(Out6) -> Out7/1
  Enabled Subsystem/7(Out7) -> Out8/1
  Enabled Subsystem/8(Out8) -> Out9/1
  S-Function/6 -> Enabled Subsystem/5(In5)
  S-Function/7 -> Enabled Subsystem/6(In6)
  S-Function/8 -> Enabled Subsystem/7(In7)
  S-Function/5 -> Enabled Subsystem/4(In4)
  S-Function/4 -> Enabled Subsystem/3(In3)
  S-Function/9 -> Enabled Subsystem/8(In8)

== system HANcoder_E407_TTA_Controller_v3/HANcoder STM32 Target - E407-STM32 algorithm/Global Ticks Increment/CAN1 Recieve/RxID_CAN/Vote2_ID_CAN/CAN receive1 ==
  In1 : Inport
  Enabled Subsystem : Subsystem  TreatAsAtomicUnit=on
  S-Function : M-S-Function  FunctionName=sfcn_can_receive  Parameters=tsamp, canBus, outputNumber, dataType, byteOrder
  Out1 : Outport
  Out2 : Outport  Port=2
  Out3 : Outport  Port=3
  Out4 : Outport  Port=4
  Out5 : Outport  Port=5
  Out6 : Outport  Port=6
  Out7 : Outport  Port=7
  Out8 : Outport  Port=8
  Out9 : Outport  Port=9
  wires:
  In1/1 -> S-Function/1
  S-Function/1 -> Enabled Subsystem/Enable, Out1/1
  S-Function/2 -> Enabled Subsystem/1(In1)
  S-Function/3 -> Enabled Subsystem/2(In2)
  Enabled Subsystem/1(Out1) -> Out2/1
  Enabled Subsystem/2(Out2) -> Out3/1
  Enabled Subsystem/3(Out3) -> Out4/1
  Enabled Subsystem/4(Out4) -> Out5/1
  Enabled Subsystem/5(Out5) -> Out6/1
  Enabled Subsystem/6(Out6) -> Out7/1
  Enabled Subsystem/7(Out7) -> Out8/1
  Enabled Subsystem/8(Out8) -> Out9/1
  S-Function/6 -> Enabled Subsystem/5(In5)
  S-Function/7 -> Enabled Subsystem/6(In6)
  S-Function/8 -> Enabled Subsystem/7(In7)
  S-Function/5 -> Enabled Subsystem/4(In4)
  S-Function/4 -> Enabled Subsystem/3(In3)
  S-Function/9 -> Enabled Subsystem/8(In8)

== system HANcoder_E407_TTA_Controller_v3/HANcoder STM32 Target - E407-STM32 algorithm/Global Ticks Increment/CAN1 Recieve/RxID_CAN/Vote3_ID_CAN/CAN receive1 ==
  In1 : Inport
  Enabled Subsystem : Subsystem  TreatAsAtomicUnit=on
  S-Function : M-S-Function  FunctionName=sfcn_can_receive  Parameters=tsamp, canBus, outputNumber, dataType, byteOrder
  Out1 : Outport
  Out2 : Outport  Port=2
  Out3 : Outport  Port=3
  Out4 : Outport  Port=4
  Out5 : Outport  Port=5
  Out6 : Outport  Port=6
  Out7 : Outport  Port=7
  Out8 : Outport  Port=8
  Out9 : Outport  Port=9
  wires:
  In1/1 -> S-Function/1
  S-Function/1 -> Enabled Subsystem/Enable, Out1/1
  S-Function/2 -> Enabled Subsystem/1(In1)
  S-Function/3 -> Enabled Subsystem/2(In2)
  Enabled Subsystem/1(Out1) -> Out2/1
  Enabled Subsystem/2(Out2) -> Out3/1
  Enabled Subsystem/3(Out3) -> Out4/1
  Enabled Subsystem/4(Out4) -> Out5/1
  Enabled Subsystem/5(Out5) -> Out6/1
  Enabled Subsystem/6(Out6) -> Out7/1
  Enabled Subsystem/7(Out7) -> Out8/1
  Enabled Subsystem/8(Out8) -> Out9/1
  S-Function/6 -> Enabled Subsystem/5(In5)
  S-Function/7 -> Enabled Subsystem/6(In6)
  S-Function/8 -> Enabled Subsystem/7(In7)
  S-Function/5 -> Enabled Subsystem/4(In4)
  S-Function/4 -> Enabled Subsystem/3(In3)
  S-Function/9 -> Enabled Subsystem/8(In8)

== system HANcoder_E407_TTA_Controller_v3/HANcoder STM32 Target - E407-STM32 algorithm/Global Ticks Increment/CAN2 Recieve/RxID_CAN/OutControl1_ID_CAN/CAN receive1 ==
  In1 : Inport
  Enabled Subsystem : Subsystem  TreatAsAtomicUnit=on
  S-Function : M-S-Function  FunctionName=sfcn_can_receive  Parameters=tsamp, canBus, outputNumber, dataType, byteOrder
  Out1 : Outport
  Out2 : Outport  Port=2
  Out3 : Outport  Port=3
  Out4 : Outport  Port=4
  Out5 : Outport  Port=5
  Out6 : Outport  Port=6
  Out7 : Outport  Port=7
  Out8 : Outport  Port=8
  Out9 : Outport  Port=9
  wires:
  S-Function/9 -> Enabled Subsystem/8(In8)
  S-Function/4 -> Enabled Subsystem/3(In3)
  S-Function/5 -> Enabled Subsystem/4(In4)
  S-Function/8 -> Enabled Subsystem/7(In7)
  S-Function/7 -> Enabled Subsystem/6(In6)
  S-Function/6 -> Enabled Subsystem/5(In5)
  Enabled Subsystem/8(Out8) -> Out9/1
  Enabled Subsystem/7(Out7) -> Out8/1
  Enabled Subsystem/6(Out6) -> Out7/1
  Enabled Subsystem/5(Out5) -> Out6/1
  Enabled Subsystem/4(Out4) -> Out5/1
  Enabled Subsystem/3(Out3) -> Out4/1
  Enabled Subsystem/2(Out2) -> Out3/1
  Enabled Subsystem/1(Out1) -> Out2/1
  S-Function/3 -> Enabled Subsystem/2(In2)
  S-Function/2 -> Enabled Subsystem/1(In1)
  S-Function/1 -> Out1/1, Enabled Subsystem/Enable
  In1/1 -> S-Function/1

== system HANcoder_E407_TTA_Controller_v3/HANcoder STM32 Target - E407-STM32 algorithm/Global Ticks Increment/CAN2 Recieve/RxID_CAN/OutControl2_ID_CAN/CAN receive1 ==
  In1 : Inport
  Enabled Subsystem : Subsystem  TreatAsAtomicUnit=on
  S-Function : M-S-Function  FunctionName=sfcn_can_receive  Parameters=tsamp, canBus, outputNumber, dataType, byteOrder
  Out1 : Outport
  Out2 : Outport  Port=2
  Out3 : Outport  Port=3
  Out4 : Outport  Port=4
  Out5 : Outport  Port=5
  Out6 : Outport  Port=6
  Out7 : Outport  Port=7
  Out8 : Outport  Port=8
  Out9 : Outport  Port=9
  wires:
  In1/1 -> S-Function/1
  S-Function/1 -> Enabled Subsystem/Enable, Out1/1
  S-Function/2 -> Enabled Subsystem/1(In1)
  S-Function/3 -> Enabled Subsystem/2(In2)
  Enabled Subsystem/1(Out1) -> Out2/1
  Enabled Subsystem/2(Out2) -> Out3/1
  Enabled Subsystem/3(Out3) -> Out4/1
  Enabled Subsystem/4(Out4) -> Out5/1
  Enabled Subsystem/5(Out5) -> Out6/1
  Enabled Subsystem/6(Out6) -> Out7/1
  Enabled Subsystem/7(Out7) -> Out8/1
  Enabled Subsystem/8(Out8) -> Out9/1
  S-Function/6 -> Enabled Subsystem/5(In5)
  S-Function/7 -> Enabled Subsystem/6(In6)
  S-Function/8 -> Enabled Subsystem/7(In7)
  S-Function/5 -> Enabled Subsystem/4(In4)
  S-Function/4 -> Enabled Subsystem/3(In3)
  S-Function/9 -> Enabled Subsystem/8(In8)

== system HANcoder_E407_TTA_Controller_v3/HANcoder STM32 Target - E407-STM32 algorithm/Global Ticks Increment/CAN2 Recieve/RxID_CAN/OutEmulator_ID_CAN/CAN receive1 ==
  In1 : Inport
  Enabled Subsystem : Subsystem  TreatAsAtomicUnit=on
  S-Function : M-S-Function  FunctionName=sfcn_can_receive  Parameters=tsamp, canBus, outputNumber, dataType, byteOrder
  Out1 : Outport
  Out2 : Outport  Port=2
  Out3 : Outport  Port=3
  Out4 : Outport  Port=4
  Out5 : Outport  Port=5
  Out6 : Outport  Port=6
  Out7 : Outport  Port=7
  Out8 : Outport  Port=8
  Out9 : Outport  Port=9
  wires:
  S-Function/9 -> Enabled Subsystem/8(In8)
  S-Function/4 -> Enabled Subsystem/3(In3)
  S-Function/5 -> Enabled Subsystem/4(In4)
  S-Function/8 -> Enabled Subsystem/7(In7)
  S-Function/7 -> Enabled Subsystem/6(In6)
  S-Function/6 -> Enabled Subsystem/5(In5)
  Enabled Subsystem/8(Out8) -> Out9/1
  Enabled Subsystem/7(Out7) -> Out8/1
  Enabled Subsystem/6(Out6) -> Out7/1
  Enabled Subsystem/5(Out5) -> Out6/1
  Enabled Subsystem/4(Out4) -> Out5/1
  Enabled Subsystem/3(Out3) -> Out4/1
  Enabled Subsystem/2(Out2) -> Out3/1
  Enabled Subsystem/1(Out1) -> Out2/1
  S-Function/3 -> Enabled Subsystem/2(In2)
  S-Function/2 -> Enabled Subsystem/1(In1)
  S-Function/1 -> Out1/1, Enabled Subsystem/Enable
  In1/1 -> S-Function/1
